simulink model "test_model"  (R2024a)
settings: Solver=VariableStepAuto  StartTime=0.0  StopTime=10.0  RelTol=1e-3
settings Model: Creator=Lenovo  LastModifiedBy=Lenovo

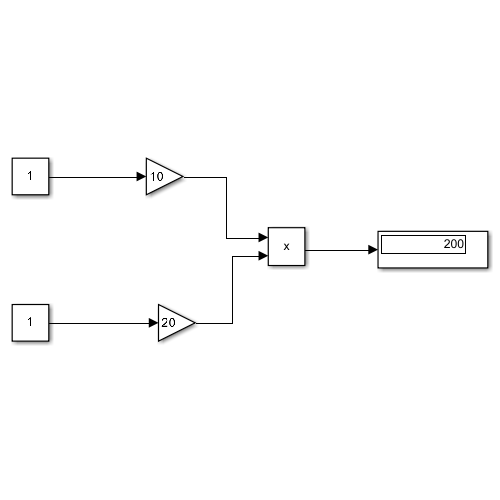
[thumbnail: Simulink's stored preview of the top-level diagram]
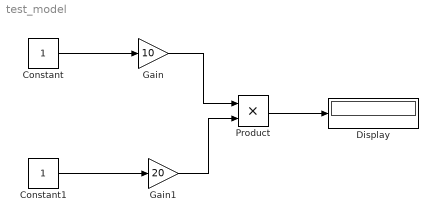
== system test_model ==
  Constant : Constant
  Constant1 : Constant
  Display : Display
  Gain : Gain  Gain=10
  Gain1 : Gain  Gain=20
  Product : Product
  wires:
  Constant/1 -> Gain/1
  Constant1/1 -> Gain1/1
  Gain/1 -> Product/1
  Gain1/1 -> Product/2
  Product/1 -> Display/1
